simulink model "DCMotorPositionControl_ClosedLoop"  (R2015b)
settings: Solver=VariableStepAuto  StartTime=0.0  StopTime=1  RelTol=1e-3
libraries: LocalLib x1
settings Model: Creator=jje  LastModifiedBy=jje

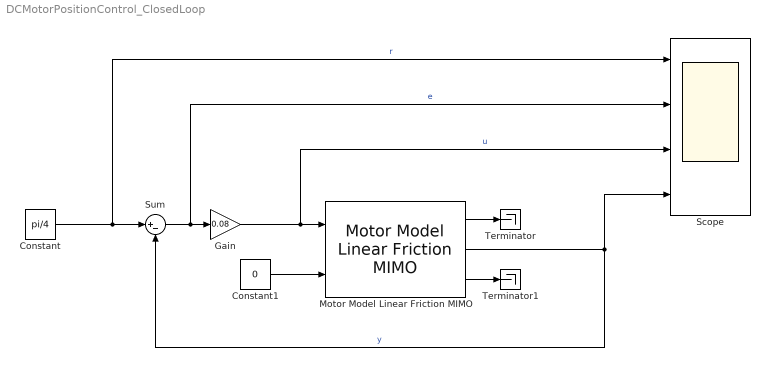
== system DCMotorPositionControl_ClosedLoop ==
  Constant : Constant  Value=pi/4
  Constant1 : Constant  Value=0
  Gain : Gain  Gain=0.08
  Motor Model Linear Friction MIMO : LocalLib/Motor Model Linear Friction MIMO
  Scope : Scope  NumInputPorts=4
  Sum : Sum  Inputs=|+-
  Terminator : Terminator
  Terminator1 : Terminator
  wires:
  Gain/1 -> Scope/3, Motor Model Linear Friction MIMO/1  "u"
  Sum/1 -> Scope/2, Gain/1  "e"
  Motor Model Linear Friction MIMO/2 -> Scope/4, Sum/2  "y"
  Constant/1 -> Scope/1, Sum/1  "r"
  Constant1/1 -> Motor Model Linear Friction MIMO/2
  Motor Model Linear Friction MIMO/1 -> Terminator/1
  Motor Model Linear Friction MIMO/3 -> Terminator1/1
